simulink model "MVB1AnyLengthThree"  (R2013b)
settings: Solver=ode45  StartTime=0.0  StopTime=6e-5  RelTol=1e-3
libraries: simulink x4
(part 2 of 2)

== stateflow chart MVB1AnyLengthThree/MVB1/redundancy ==
  note: 从上一个接收事件后总线寂静1.4ms则产生一总线寂静的通知
  state Timer1 [parallel]
    settings: executionOrder=1
    state Timer
    state start
    state TimeOut
      entry:
      trust = false;
    Timer1.start -> Timer1.Timer : [judge(MFReceive1, MFReceive2, SFReceive1, SFReceive2, trust) == false]
        | {
        | t1 = clock_Counter;
        | }
    (default) -> Timer1.start
    Timer1.Timer -> Timer1.start [order 1] : [judge(MFReceive1, MFReceive2, SFReceive1, SFReceive2, trust) == true]
    Timer1.TimeOut -> Timer1.start
    Timer1.Timer -> Timer1.TimeOut [order 2] : [clock_Counter - t1 > (1400/prop) && judge(MFReceive1, MFReceive2, SFReceive1, SFReceive2, trust) == false]
  note: 上一个主帧接收后1.3ms没有收到主帧产生一个主帧超时的通知。
  state Timer2 [parallel]
    settings: executionOrder=2
    state Timer
    state start
    state TimeOut
      entry:
      trust = false;
    Timer2.start -> Timer2.Timer : [judge(MFReceive1, MFReceive2, trust) == true]
        | {
        | t1 = clock_Counter;
        | }
    (default) -> Timer2.start
    Timer2.Timer -> Timer2.start [order 1] : [judge(MFReceive1, MFReceive2,  trust) == true]
    Timer2.TimeOut -> Timer2.start
    Timer2.Timer -> Timer2.TimeOut [order 2] : [clock_Counter - t1 > (1300/prop) && judge(MFReceive1, MFReceive2,  trust) == false]
  note: 收到主帧后42.7us没有收到从帧产生从帧超时的通知。
  state Timer3 [parallel]
    settings: executionOrder=3
    state Timer
    state start
    state TimeOut
      entry:
      trust = false;
    Timer3.start -> Timer3.Timer : [judge(MFReceive1, MFReceive2, trust) == true]
        | {
        | t1 = clock_Counter;
        | }
    (default) -> Timer3.start
    Timer3.Timer -> Timer3.start [order 1] : [judge(SFReceive1, SFReceive2, trust) == true]
    Timer3.TimeOut -> Timer3.start
    Timer3.Timer -> Timer3.TimeOut [order 2] : [clock_Counter - t1 > (42.7/prop) && judge(SFReceive1, SFReceive2, trust) == false]
  note: 信任线未收到数据，而观察线收到数据时切换
  state observer [parallel]
    settings: executionOrder=4
    state A
      entry:
      trust = true;
    state B
      entry:
      trust = false;
    observer.A -> observer.B : [judge(MFReceive1, MFReceive2, SFReceive1, SFReceive2, trust) == false]
    (default) -> observer.A
    observer.B -> observer.A : [judge(MFReceive1, MFReceive2, SFReceive1, SFReceive2, trust) == true]
  state trans [parallel]
    settings: executionOrder=5
    state B
      during:
      MFReceive = MFReceive2;
      MFIn = MFIn2;
      SFReceive = SFReceive2;
      SFIn = SFIn2;
    state A
      during:
      MFReceive = MFReceive1;
      MFIn = MFIn1;
      SFReceive = SFReceive1;
      SFIn = SFIn1;
    trans.A -> trans.B : [trust == false]
        | {
        | MFReceive = MFReceive2;
        | MFIn = MFIn2;
        | SFReceive = SFReceive2;
        | SFIn = SFIn2;
        | }
    trans.B -> trans.A : [trust == true]
        | {
        | MFReceive = MFReceive1;
        | MFIn = MFIn1;
        | SFReceive = SFReceive1;
        | SFIn = SFIn1;
        | }
    (default) -> trans.A
  data: r function_output boolean; m1 function_input boolean; m2 function_input boolean; s1 function_input boolean; s2 function_input boolean; t function_input boolean; r function_output boolean; m1 function_input boolean; m2 function_input boolean; t function_input boolean; r function_output boolean; m1 function_input boolean; m2 function_input boolean; t function_input boolean; r function_output boolean; s1 function_input boolean; s2 function_input boolean; t function_input boolean; r function_output boolean; m1 function_input boolean; m2 function_input boolean; s1 function_input boolean; s2 function_input boolean; t function_input boolean; MFReceive1 input boolean; SFReceive1 input boolean; MFIn1 input uint32; SFIn1 input uint32; MFReceive2 input boolean; SFReceive2 input boolean; MFIn2 input uint32; SFIn2 input uint32; MFReceive output boolean; SFReceive output boolean; MFIn output uint32; SFIn output uint32; t1 local uint32; clock_Counter data_store_memory; trust local boolean =true; prop data_store_memory
  function r = judge(m1, m2, s1, s2, t):
    | function r = judge(m1, m2, s1, s2, t)
    | r = true;
    | if t == true
    |     if m1||s1 == false
    |         r = false;
    |     end
    | else
    |     if m2||s2 == false
    |         r = false;
    |     end
    | end
  function r = judge(m1, m2,t):
    | function r = judge(m1, m2,t)
    | r = false;
    | if t == true
    |     if m1 == true
    |         r = true;
    |     end
    | else
    |     if m2 == true
    |         r = true;
    |     end
    | end
  function r = judge(m1, m2, t):
    | function r = judge(m1, m2, t)
    | r = false;
    | if t == true
    |     if m1 == true
    |         r = true;
    |     end
    | else
    |     if m2 == true
    |         r = true;
    |     end
    | end
  function r = judgeSF(s1, s2, t):
    | function r = judgeSF(s1, s2, t)
    | r = false;
    | if t == true
    |     if s1 == true
    |         r = true;
    |     end
    | else
    |     if s2 == true
    |         r = true;
    |     end
    | end
  function r = judge(m1, m2, s1, s2, t):
    | function r = judge(m1, m2, s1, s2, t)
    | r = true;
    | if t == true
    |     if (m1||s1 == false) && (m2||s2 == true)
    |         r = false;
    |     end
    | else
    |     if (m2||s2 == false) && (m1||s1 == true)
    |         r = false;
    |     end
    | end

== stateflow chart MVB1AnyLengthThree/MVB3/Subsystem/Decoder ==
  state decodeSF
    decodeSF -> decodeSF [order 1] : CLK
        | {
        | ans = bitoperate.shiftbit(ans, 1) + SFIn;
        | count++;
        | }
  state bitoperate [group]
  state judge
    entry:
    ans = 0;
  state start
  state decodeMF
    decodeMF -> decodeMF [order 1] : CLK
        | {
        | ans = bitoperate.shiftbit(ans, 1) + MFIn;
        | count++;
        | }
  decodeSF -> judge [order 1] : [count==32]
      | {
      | SDataOut = ManchesterDecoding(ans);
      | count=0;
      | SFBuffer[SFBufferIndex] = SDataOut;
      | SFBufferIndex++;
      | }
  start -> decodeSF [order 2] : [SFInSign == true]
      | {
      | ans = 0;
      | count = 1;
      | SDataOut = 0;
      | ans = bitoperate.shiftbit(ans, 1) + SFIn;
      | SOutSign = true;
      | }
  judge -> decodeSF [order 1] : [SFInSign==true]
  judge -> start [order 2] : {
      | SOutSign = false;
      | SDataOut = 0;
      | }
  start -> decodeMF [order 1] : [MFInSign==true]
      | {
      | ans = 0;
      | count = 0;
      | MDataOut = 0;
      | MOutSign = true
      | ans = bitoperate.shiftbit(ans, 1) + MFIn;
      | count++;
      | }
  (default) -> start
  decodeMF -> start [order 1] : [count==32]
      | {
      | ans = ManchesterDecoding(ans);
      | MDataOut = ans;
      | MOutSign = false;
      | }
  data: num function_input uint32; r function_output uint32; data function_input uint32; num function_input uint32; r function_output uint32; r function_output uint32; data function_input uint32; MFIn input uint32; SFIn input uint32; MDataOut output uint32; MFInSign input boolean; count local uint32; SFInSign input boolean; SDataOut output uint32; MOutSign output boolean; SOutSign output boolean; ans local uint32; SFBuffer data_store_memory; SFBufferIndex data_store_memory
  events: CLK input EITHER_EDGE_EVENT
  function r = getbit(num):
    | function r = getbit(num)
    | r = bitget(num, 32);
  function r = shiftbit(data, num):
    | function r = shiftbit(data, num)
    | r = bitshift(data, num);
    | %for i=1:cnt
    | %   r = bitset(r, i, 0);
    | %end
  function r = ManchesterDecoding(data):
    | function r = ManchesterDecoding(data)
    | r = uint32(0);
    | for i = (1:2:32)
    |     x0 = bitget(data, i);
    |     x1 = bitget(data, i+1);
    |     if x0==0 && x1==1
    |         r = bitset(r, (i+1)/2, 1);
    |     else
    |         r = bitset(r, (i+1)/2, 0);
    |     end
    | end

== stateflow chart MVB1AnyLengthThree/MVB3/Subsystem/MainProc ==
  note: 上一个主帧接收后1.3ms没有收到主帧产生一个主帧超时的通知。
  state Timer [parallel]
    settings: executionOrder=1
    state Timer
      entry:
      t = clock_Counter;
      timeOut = false;
    state start
    state TimeOut
      entry:
      timeOut = true;
    start -> Timer.Timer : [startTimer == true]
    (default) -> start
    Timer.Timer -> start [order 1] : [endTimer == true]
    Timer.TimeOut -> start
    Timer.Timer -> Timer.TimeOut [order 2] : [clock_Counter - t > (1300/prop)]
  state mainproc [parallel]
    settings: executionOrder=2
    state StandbyEquip
      entry:
      startTimer = true;
      endTimer = false;
    state MainEquip
    state TimeOut
    state wait4ACT
    note: 等待其他设备返回ACT
    note: 等待其他设备返回OK，receiver在接收到OK以后立马放弃主权
    state TempEquip
      entry:
      startTimer = true;
      endTimer = false;
    (default) -> StandbyEquip
    mainproc.TimeOut -> StandbyEquip
    StandbyEquip -> mainproc.TimeOut [order 2] : [timeOut == true]
    TempEquip -> StandbyEquip [order 1] : [BA == false]
        | {
        | endTimer = true;
        | startTimer = false;
        | }
    StandbyEquip -> MainEquip [order 1] : [BA == true && ACT == true]
        | {
        | endTimer = true;
        | startTimer = false;
        | }
    MainEquip -> wait4ACT : [acceptACT == true]
        | {
        | t = clock_Counter;
        | }
    TempEquip -> mainproc.TimeOut [order 2] : [timeOut == true]
    wait4ACT -> TempEquip : [acceptDomain == true]
        | {
        | t = clock_Counter;
        | }
  data: BA data_store_memory; ACT local boolean =true; acceptACT data_store_memory; acceptDomain data_store_memory; t local uint32; clock_Counter data_store_memory; startTimer local boolean; timeOut local boolean; endTimer local boolean; prop data_store_memory

== stateflow chart MVB1AnyLengthThree/MVB2/Subsystem/Sender ==
  state SFSender [parallel]
    settings: executionOrder=1
    note: send**Signd的置位在接收到了请求数据的主帧后置位
    state sender [parallel]
      settings: executionOrder=1
      state wait
      state sendInfo
      state sendRandomSF
      state sendOK
      state transmission
        entry:
        SOutSign = true;
      (default) -> SFSender.sender.wait
      SFSender.sender.wait -> sendRandomSF [order 1] : [sendRandSFSign == true]
      SFSender.sender.wait -> sendOK [order 2] : [sendOkSign == true]
          | {
          | isMaster = true;
          | }
      SFSender.sender.wait -> sendInfo [order 3] : [sendACTSign == true]
      sendInfo -> SFSender.sender.transmission : {SFIndex = 1;
          | sendACTSign = false;}
      sendRandomSF -> SFSender.sender.transmission : {SFIndex = 0;
          | sendRandSFSign = false;}
      sendOK -> SFSender.sender.transmission : {SFIndex = 2;
          | sendOkSign = false;
          | init();
          | BA = true;
          | }
      SFSender.sender.transmission -> SFSender.sender : SFTransDone
          | {SDataOut = uint32(0);
          | SOutSign = false;
          | }
    state sendHolder [parallel]
      settings: executionOrder=2
      state judge
      state full
        SFSender.sendHolder.full -> SFSender.sendHolder.full [order 1] : CLK
            | {
            | SDataOut = bitoperate.getbit(input);
            | input = bitoperate.shiftbit(input, uint32(1));
            | count = count + 1;
            | }
      state empty
      judge -> SFSender.sendHolder.empty [order 2] : {
          | SOutSign = false;
          | SFCurrentIndex = 2;
          | send(SFTransDone, sender);
          | }
      SFSender.sendHolder.full -> judge [order 1] : [count == 32]
          | {
          | SFCurrentIndex = SFCurrentIndex + 1;
          | }
      judge -> SFSender.sendHolder.full [order 1] : [SFCurrentIndex <= SFT(SFIndex*16 + 1)]
          | {
          | input = ManchesterEncoding(uint32(SFT(SFIndex*16+SFCurrentIndex)));
          | count = 0;
          | }
      (default) -> SFSender.sendHolder.empty : {
          | SFCurrentIndex = 2;
          | }
      SFSender.sendHolder.empty -> SFSender.sendHolder.full : enter(sender.transmission)
          | {
          | input = ManchesterEncoding(uint32(SFT(SFIndex*16+SFCurrentIndex)));
          | SOutSign = true;
          | SDataOut = uint32(0);
          | count = 0;
          | }
  state MFSender [parallel]
    settings: executionOrder=2
    state sender [parallel]
      settings: executionOrder=1
      state sleep
      state wait
        entry:
        signal1 = true
      state transmission
        entry:
        signal1 = false;
        MOutSign = true;
        [acceptSF, acceptACT, acceptDomain] = setAcceptSignal(MFT(MFIndex));
      (default) -> sleep : {
          | init();
          | }
      sleep -> MFSender.sender.wait : CLK_3M
          | [BA==true ]
      MFSender.sender.transmission -> sleep : exit(buffer.full)
          | {
          | MDataOut = uint32(0);
          | MOutSign = false;
          | MFIndex = MFIndex + 1;
          | }
      MFSender.sender.wait -> MFSender.sender.transmission : [trans1 == true]
    state buffer [parallel]
      settings: executionOrder=2
      state full
        entry:
        count = 0;
        MFSender.buffer.full -> MFSender.buffer.full [order 1] : CLK
            | {
            | MDataOut = bitoperate.getbit(input);
            | input = bitoperate.shiftbit(input, uint32(1));
            | count = count + 1;
            | }
      state empty
      (default) -> MFSender.buffer.empty
      MFSender.buffer.full -> MFSender.buffer.empty [order 1] : [count == 32]
      MFSender.buffer.empty -> MFSender.buffer.full : enter(sender.transmission)
          | {
          | input =  ManchesterEncoding(MFT(MFIndex));
          | count = 0;
          | }
  state init [function]
    note: 请求随机从帧
        | 请求随机从帧
        | 请求2号的信息
        | 请求转移到2号
    note: SFT(1)代表随机的从帧
        | SFT(2)代表回复接受主权
        | SFT(3)代表回复设备ACT和BA
    (default) -> (junction 100) : {
        | BA = false;
        | MFIndex = 1;
        | isMaster = false;
        | SendSignal = false;
        | MFT(1) = getMF(0, 1);
        | MFT(2) = getMF(0, 3);
        | MFT(3) = getMF(8, 3);
        | MFT(4) = getMF(15, 3);
        | MFT(5) = 1;
        | SFT(1) = 4;
        | SFT(2) = 10894;
        | SFT(3) = 12428;
        | SFT(4) = 19;
        | SFT(17) = 4;
        | SFT(18) = 10894;
        | SFT(19) = 12832;
        | SFT(20) = 3;
        | SFT(33) = 4;
        | SFT(34) = 10894;
        | SFT(35) = 14464;
        | SFT(36) = 3;
        | clock_3M_shang = false;
        | sendRandSFSign = false;
        | sendACTSign = false;
        | sendRandSFSign = false;
        | }
  state bitoperate [group]
  (default) -> MFSender
  data: SFCurrentIndex local double; count local double; input local uint32; SFIndex local double; dataIn function_input uint32; SF function_output boolean; ACT function_output; Domain function_output; input local uint32; count local double; data function_input uint32; r function_output uint32; f_code function_input; addr function_input; r function_output; addr function_input; r function_output; r function_output uint32; data function_input uint32; num function_input uint32; r function_output uint32; data function_input uint32; num function_input uint32; r function_output uint32; MFReceive input boolean; MDataOut output uint32; clock_3M data_store_memory; clock_Counter data_store_memory; MFIndex local; MFT local uint32 size=5; trans1 data_store_memory; signal1 data_store_memory; SFReceive input boolean; sendOkSign data_store_memory; sendRandSFSign data_store_memory; sendACTSign data_store_memory; SDataOut output uint32; MOutSign output boolean; SOutSign output boolean; isMaster local boolean; acceptSF data_store_memory; BA data_store_memory; clock_3M_shang local boolean; acceptACT data_store_memory; acceptDomain data_store_memory; prop data_store_memory; SFT local uint16 size=100
  events: SFTransDone local FUNCTION_CALL_EVENT; CLK input EITHER_EDGE_EVENT; CLK_3M input EITHER_EDGE_EVENT
  function judgeMaster:
    | function judgeMaster
    | % 如果
    | if isMaster == true && SFIndex == 2
    |     isMaster = false;
    | end
  function [SF, ACT, Domain] = setAcceptSignal(dataIn):
    | function [SF, ACT, Domain] = setAcceptSignal(dataIn)
    | % 右移12位 仅保留帧头和fcode
    | dataInExAddr = bitshift(uint32(dataIn), -12);
    | % 先右移16位再左移4位 仅仅保留帧头
    | dataInStart = bitshift(bitshift(uint32(dataIn), -16), 4);
    | % 相减得到fcode
    | fcode = double(dataInExAddr - dataInStart);
    | SF = false;
    | Domain = false;
    | ACT = false;
    | if fcode == 0
    |     SF = true;
    | elseif fcode == 8
    |     ACT = true;
    | else
    |     Domain = true;
    | end
  function r = ManchesterEncoding(data):
    | function r = ManchesterEncoding(data)
    | r = data;
    | for i = 1:16
    |     x = bitget(data, i);
    |     if x == 0
    |         r = bitset(r, i*2-1, 1);
    |         r = bitset(r, i*2, 0);
    |     else
    |         r = bitset(r, i*2-1, 0);
    |         r = bitset(r, i*2, 1);
    |     end
    | end
  function r = getMF(f_code, addr):
    | function r = getMF(f_code, addr)
    | r = 3340042240;
    | r = r + bitshift(uint32(f_code), 12);
    | r = r + addr;
  function r = getSF(addr):
    | function r = getSF(addr)
    | r = 2833448960;
    | r = r + addr;
  function r = ManchesterDecoding(data):
    | function r = ManchesterDecoding(data)
    | r = uint32(0);
    | for i = (1:2:32)
    |     x0 = bitget(data, i);
    |     x1 = bitget(data, i+1);
    |     if x0==0 && x1==1
    |         r = bitset(r, (i+1)/2, 1);
    |     else
    |         r = bitset(r, (i+1)/2, 0);
    |     end
    | end
  function r = getbit(num):
    | function r = getbit(num)
    | r = bitget(num, 32);
  function r = shiftbit(data, num):
    | function r = shiftbit(data, num)
    | r = bitshift(data, num);
    | %for i=1:cnt
    | %   r = bitset(r, i, 0);
    | %end

== stateflow chart MVB1AnyLengthThree/MVB3/Subsystem/Receiver ==
  state receiveMF [parallel]
    settings: executionOrder=1
    state wait
    state wait4MFEnd
    state judgeAddr
    state MFReceive
    state MFcode0
    state MFcode8
    state MFcode15
    state MTrans
    (default) -> receiveMF.wait : {
        | t = clock_Counter;
        | }
    judgeAddr -> receiveMF.wait [order 2]
    MTrans -> receiveMF.wait : [sendRandSFSign == false && sendOkSign == false && sendACTSign == false]
        | {
        | t = clock_Counter;
        | }
    receiveMF.wait -> wait4MFEnd : [MFReceive==true]
    wait4MFEnd -> judgeAddr : [MFReceive == false]
        | {fcodeIn = uint8(getFCode(MFIn));
        | addrIn = uint16(getAddr(MFIn));
        | t = 0;
        | }
    judgeAddr -> MFReceive [order 1] : [addrIn == LogicAddr]
    MFReceive -> MFcode0 [order 2] : [fcodeIn == 0 && MFReceive == false ]
    MFReceive -> MFcode8 [order 3] : [fcodeIn == 8 && MFReceive == false]
    MFReceive -> MFcode15 [order 1] : [fcodeIn == 15 && MFReceive == false]
    MFcode0 -> MTrans : {sendRandSFSign = true}
    MFcode8 -> MTrans : {sendACTSign = true}
    MFcode15 -> MTrans : {sendOkSign = true}
  state receiveSF [parallel]
    settings: executionOrder=2
    note: acceptSF, acceptACT, acceptDomain在发送完主帧以后，根据主帧的类型进行相应的置位
        | 收到fcode为8的从帧之后，说明目标设备已经返回了OK，这时应该将ismaster设为1
    state wait
    state wait4SFEnd
    state judge4SF
    state wait4SF
    state wait4ACT
    state wait4Domain
    state STrans
    (default) -> receiveSF.wait
    (junction 96) -> receiveSF.wait : {
        | SFBufferIndex = 0;
        | initSFBuffer();
        | }
    receiveSF.wait -> wait4SFEnd : [SFReceive == true]
        | {
        | t = 0;
        | }
    wait4SFEnd -> judge4SF : [SFReceive == false]
    judge4SF -> (junction 96) [order 4]
    STrans -> (junction 96) : [SFReceive == false]
    judge4SF -> wait4Domain [order 3] : [acceptDomain == true]
    judge4SF -> wait4SF [order 1] : [acceptSF == true]
    judge4SF -> wait4ACT [order 2] : [acceptACT == true]
    wait4SF -> STrans : {
        | acceptSF = false;
        | }
    wait4ACT -> STrans : [getbit(SFBuffer[1], 6)]
        | {
        | acceptACT = false;
        | }
    wait4Domain -> STrans : [getbit(SFBuffer[1], 8) == 1]
        | {
        | acceptDomain = false;
        | BA = false;
        | }
  state initSFBuffer [function]
    (default) -> (junction 157) : /* init SFBuffer */
    (junction 149) -> (junction 151) [order 1] : [index<16]
    (junction 151) -> (junction 148) : {SFBuffer[index] = 0;}
    (junction 157) -> (junction 149) : {index=0;}
    (junction 148) -> (junction 149) : {index++;}
    (junction 149) -> (junction 145) [order 2]
  note: SFBufferIndex需要在每次读取后清零
  note: 期待目标设备返回OK
  data: index local double; dataIn function_input uint32; num function_input uint32; r function_output uint32; dataIn function_input double; r function_output double; data function_input uint32; r function_output uint32; dataIn function_input double; r function_output double; r function_output uint32; data function_input uint32; MFIn input uint32; SFIn input uint32; t local uint32; clock_Counter data_store_memory; clock_3M data_store_memory; MFReceive input boolean; SFReceive input boolean; fcodeIn local uint8; addrIn local uint16; trans1 data_store_memory; LogicAddr data_store_memory; sendRandSFSign data_store_memory; sendOkSign data_store_memory; sendACTSign data_store_memory; acceptSF data_store_memory; acceptDomain data_store_memory; acceptACT data_store_memory; BA data_store_memory; SFBuffer data_store_memory; SFBufferIndex data_store_memory
  function r = getbit(dataIn, num):
    | function r = getbit(dataIn, num)
    | r = bitget(uint32(dataIn), num);
  function r = getFCode(dataIn):
    | function r = getFCode(dataIn)
    | % 右移12位 仅保留帧头和fcode
    | dataInExAddr = bitshift(uint32(dataIn), -12);
    | % 先右移16位再左移4位 仅仅保留帧头
    | dataInStart = bitshift(bitshift(uint32(dataIn), -16), 4);
    | % 相减得到fcode
    | r = double(dataInExAddr - dataInStart);
  function r = ManchesterEncoding(data):
    | function r = ManchesterEncoding(data)
    | r = data;
    | for i = 1:16
    |     x = bitget(data, i);
    |     if x == 0
    |         r = bitset(r, i*2-1, 1);
    |         r = bitset(r, i*2, 0);
    |     else
    |         r = bitset(r, i*2-1, 0);
    |         r = bitset(r, i*2, 1);
    |     end
    | end
  function r = getAddr(dataIn):
    | function r = getAddr(dataIn)
    | % 把后12位也就是地址归零
    | dataInExAddr = bitshift(bitshift(uint32(dataIn), -12), 12);
    | % 相减获取地址
    | r = double(dataIn - dataInExAddr);
  function r = ManchesterDecoding(data):
    | function r = ManchesterDecoding(data)
    | r = uint32(0);
    | for i = (1:2:32)
    |     x0 = bitget(data, i);
    |     x1 = bitget(data, i+1);
    |     if x0==0 && x1==1
    |         r = bitset(r, (i+1)/2, 1);
    |     else
    |         r = bitset(r, (i+1)/2, 0);
    |     end
    | end

== stateflow chart MVB1AnyLengthThree/MVB3/Subsystem/Sender ==
  state SFSender [parallel]
    settings: executionOrder=1
    note: send**Signd的置位在接收到了请求数据的主帧后置位
    state sender [parallel]
      settings: executionOrder=1
      state wait
      state sendInfo
      state sendRandomSF
      state sendOK
      state transmission
        entry:
        SOutSign = true;
      (default) -> SFSender.sender.wait
      SFSender.sender.wait -> sendRandomSF [order 1] : [sendRandSFSign == true]
      SFSender.sender.wait -> sendOK [order 2] : [sendOkSign == true]
          | {
          | isMaster = true;
          | }
      SFSender.sender.wait -> sendInfo [order 3] : [sendACTSign == true]
      sendInfo -> SFSender.sender.transmission : {SFIndex = 1;
          | sendACTSign = false;}
      sendRandomSF -> SFSender.sender.transmission : {SFIndex = 0;
          | sendRandSFSign = false;}
      sendOK -> SFSender.sender.transmission : {SFIndex = 2;
          | sendOkSign = false;
          | init();
          | BA = true;
          | }
      SFSender.sender.transmission -> SFSender.sender : SFTransDone
          | {SDataOut = uint32(0);
          | SOutSign = false;
          | }
    state sendHolder [parallel]
      settings: executionOrder=2
      state judge
      state full
        SFSender.sendHolder.full -> SFSender.sendHolder.full [order 1] : CLK
            | {
            | SDataOut = bitoperate.getbit(input);
            | input = bitoperate.shiftbit(input, uint32(1));
            | count = count + 1;
            | }
      state empty
      judge -> SFSender.sendHolder.empty [order 2] : {
          | SOutSign = false;
          | SFCurrentIndex = 2;
          | send(SFTransDone, sender);
          | }
      SFSender.sendHolder.full -> judge [order 1] : [count == 32]
          | {
          | SFCurrentIndex = SFCurrentIndex + 1;
          | }
      judge -> SFSender.sendHolder.full [order 1] : [SFCurrentIndex <= SFT(SFIndex*16 + 1)]
          | {
          | input = ManchesterEncoding(uint32(SFT(SFIndex*16+SFCurrentIndex)));
          | count = 0;
          | }
      (default) -> SFSender.sendHolder.empty : {
          | SFCurrentIndex = 2;
          | }
      SFSender.sendHolder.empty -> SFSender.sendHolder.full : enter(sender.transmission)
          | {
          | input = ManchesterEncoding(uint32(SFT(SFIndex*16+SFCurrentIndex)));
          | SOutSign = true;
          | SDataOut = uint32(0);
          | count = 0;
          | }
  state MFSender [parallel]
    settings: executionOrder=2
    state sender [parallel]
      settings: executionOrder=1
      state sleep
      state wait
        entry:
        signal1 = true
      state transmission
        entry:
        signal1 = false;
        MOutSign = true;
        [acceptSF, acceptACT, acceptDomain] = setAcceptSignal(MFT(MFIndex));
      (default) -> sleep : {
          | init();
          | }
      sleep -> MFSender.sender.wait : CLK_3M
          | [BA==true]
      MFSender.sender.transmission -> sleep : exit(buffer.full)
          | {
          | MDataOut = uint32(0);
          | MOutSign = false;
          | MFIndex = MFIndex + 1;
          | }
      MFSender.sender.wait -> MFSender.sender.transmission : [trans1 == true]
    state buffer [parallel]
      settings: executionOrder=2
      state full
        entry:
        count = 0;
        MFSender.buffer.full -> MFSender.buffer.full [order 1] : CLK
            | {
            | MDataOut = bitoperate.getbit(input);
            | input = bitoperate.shiftbit(input, uint32(1));
            | count = count + 1;
            | }
      state empty
      (default) -> MFSender.buffer.empty
      MFSender.buffer.full -> MFSender.buffer.empty [order 1] : [count == 32]
      MFSender.buffer.empty -> MFSender.buffer.full : enter(sender.transmission)
          | {
          | input =  ManchesterEncoding(MFT(MFIndex));
          | count = 0;
          | }
  state init [function]
    note: 请求随机从帧
        | 请求随机从帧
        | 请求2号的信息
        | 请求转移到2号
    note: SFT(1)代表随机的从帧
        | SFT(2)代表回复接受主权
        | SFT(3)代表回复设备ACT和BA
    (default) -> (junction 100) : {
        | BA = false;
        | MFIndex = 1;
        | isMaster = false;
        | SendSignal = false;
        | MFT(1) = getMF(0, 1);
        | MFT(2) = getMF(0, 2);
        | MFT(3) = getMF(8, 1);
        | MFT(4) = getMF(15, 1);
        | MFT(5) = 1;
        | SFT(1) = 4;
        | SFT(2) = 10894;
        | SFT(3) = 12428;
        | SFT(4) = 19;
        | SFT(17) = 4;
        | SFT(18) = 10894;
        | SFT(19) = 12832;
        | SFT(20) = 3;
        | SFT(33) = 4;
        | SFT(34) = 10894;
        | SFT(35) = 14464;
        | SFT(36) = 3;
        | clock_3M_shang = false;
        | sendRandSFSign = false;
        | sendACTSign = false;
        | sendRandSFSign = false;
        | }
  state bitoperate [group]
  (default) -> MFSender
  data: SFCurrentIndex local double; count local double; input local uint32; SFIndex local double; dataIn function_input uint32; SF function_output boolean; ACT function_output; Domain function_output; input local uint32; count local double; data function_input uint32; r function_output uint32; f_code function_input; addr function_input; r function_output; addr function_input; r function_output; r function_output uint32; data function_input uint32; num function_input uint32; r function_output uint32; data function_input uint32; num function_input uint32; r function_output uint32; MFReceive input boolean; MDataOut output uint32; clock_3M data_store_memory; clock_Counter data_store_memory; MFIndex local; MFT local uint32 size=5; trans1 data_store_memory; signal1 data_store_memory; SFReceive input boolean; sendOkSign data_store_memory; sendRandSFSign data_store_memory; sendACTSign data_store_memory; SDataOut output uint32; MOutSign output boolean; SOutSign output boolean; isMaster local boolean; acceptSF data_store_memory; BA data_store_memory; clock_3M_shang local boolean; acceptACT data_store_memory; acceptDomain data_store_memory; prop data_store_memory; SFT local uint16 size=100
  events: SFTransDone local FUNCTION_CALL_EVENT; CLK input EITHER_EDGE_EVENT; CLK_3M input EITHER_EDGE_EVENT
  function judgeMaster:
    | function judgeMaster
    | % 如果
    | if isMaster == true && SFIndex == 2
    |     isMaster = false;
    | end
  function [SF, ACT, Domain] = setAcceptSignal(dataIn):
    | function [SF, ACT, Domain] = setAcceptSignal(dataIn)
    | % 右移12位 仅保留帧头和fcode
    | dataInExAddr = bitshift(uint32(dataIn), -12);
    | % 先右移16位再左移4位 仅仅保留帧头
    | dataInStart = bitshift(bitshift(uint32(dataIn), -16), 4);
    | % 相减得到fcode
    | fcode = double(dataInExAddr - dataInStart);
    | SF = false;
    | Domain = false;
    | ACT = false;
    | if fcode == 0
    |     SF = true;
    | elseif fcode == 8
    |     ACT = true;
    | else
    |     Domain = true;
    | end
  function r = ManchesterEncoding(data):
    | function r = ManchesterEncoding(data)
    | r = data;
    | for i = 1:16
    |     x = bitget(data, i);
    |     if x == 0
    |         r = bitset(r, i*2-1, 1);
    |         r = bitset(r, i*2, 0);
    |     else
    |         r = bitset(r, i*2-1, 0);
    |         r = bitset(r, i*2, 1);
    |     end
    | end
  function r = getMF(f_code, addr):
    | function r = getMF(f_code, addr)
    | r = 3340042240;
    | r = r + bitshift(uint32(f_code), 12);
    | r = r + addr;
  function r = getSF(addr):
    | function r = getSF(addr)
    | r = 2833448960;
    | r = r + addr;
  function r = ManchesterDecoding(data):
    | function r = ManchesterDecoding(data)
    | r = uint32(0);
    | for i = (1:2:32)
    |     x0 = bitget(data, i);
    |     x1 = bitget(data, i+1);
    |     if x0==0 && x1==1
    |         r = bitset(r, (i+1)/2, 1);
    |     else
    |         r = bitset(r, (i+1)/2, 0);
    |     end
    | end
  function r = getbit(num):
    | function r = getbit(num)
    | r = bitget(num, 32);
  function r = shiftbit(data, num):
    | function r = shiftbit(data, num)
    | r = bitshift(data, num);
    | %for i=1:cnt
    | %   r = bitset(r, i, 0);
    | %end

== stateflow chart MVB1AnyLengthThree/MVB2/redundancy ==
  note: 从上一个接收事件后总线寂静1.4ms则产生一总线寂静的通知
  state Timer1 [parallel]
    settings: executionOrder=1
    state Timer
    state start
    state TimeOut
      entry:
      trust = false;
    Timer1.start -> Timer1.Timer : [judge(MFReceive1, MFReceive2, SFReceive1, SFReceive2, trust) == false]
        | {
        | t1 = clock_Counter;
        | }
    (default) -> Timer1.start
    Timer1.Timer -> Timer1.start [order 1] : [judge(MFReceive1, MFReceive2, SFReceive1, SFReceive2, trust) == true]
    Timer1.TimeOut -> Timer1.start
    Timer1.Timer -> Timer1.TimeOut [order 2] : [clock_Counter - t1 > (1400/prop) && judge(MFReceive1, MFReceive2, SFReceive1, SFReceive2, trust) == false]
  note: 上一个主帧接收后1.3ms没有收到主帧产生一个主帧超时的通知。
  state Timer2 [parallel]
    settings: executionOrder=2
    state Timer
    state start
    state TimeOut
      entry:
      trust = false;
    Timer2.start -> Timer2.Timer : [judge(MFReceive1, MFReceive2, trust) == true]
        | {
        | t1 = clock_Counter;
        | }
    (default) -> Timer2.start
    Timer2.Timer -> Timer2.start [order 1] : [judge(MFReceive1, MFReceive2,  trust) == true]
    Timer2.TimeOut -> Timer2.start
    Timer2.Timer -> Timer2.TimeOut [order 2] : [clock_Counter - t1 > (1300/prop) && judge(MFReceive1, MFReceive2,  trust) == false]
  note: 收到主帧后42.7us没有收到从帧产生从帧超时的通知。
  state Timer3 [parallel]
    settings: executionOrder=3
    state Timer
    state start
    state TimeOut
      entry:
      trust = false;
    Timer3.start -> Timer3.Timer : [judge(MFReceive1, MFReceive2, trust) == true]
        | {
        | t1 = clock_Counter;
        | }
    (default) -> Timer3.start
    Timer3.Timer -> Timer3.start [order 1] : [judge(SFReceive1, SFReceive2, trust) == true]
    Timer3.TimeOut -> Timer3.start
    Timer3.Timer -> Timer3.TimeOut [order 2] : [clock_Counter - t1 > (42.7/prop) && judge(SFReceive1, SFReceive2, trust) == false]
  note: 信任线未收到数据，而观察线收到数据时切换
  state observer [parallel]
    settings: executionOrder=4
    state A
      entry:
      trust = true;
    state B
      entry:
      trust = false;
    observer.A -> observer.B : [judge(MFReceive1, MFReceive2, SFReceive1, SFReceive2, trust) == false]
    (default) -> observer.A
    observer.B -> observer.A : [judge(MFReceive1, MFReceive2, SFReceive1, SFReceive2, trust) == true]
  state trans [parallel]
    settings: executionOrder=5
    state B
      during:
      MFReceive = MFReceive2;
      MFIn = MFIn2;
      SFReceive = SFReceive2;
      SFIn = SFIn2;
    state A
      during:
      MFReceive = MFReceive1;
      MFIn = MFIn1;
      SFReceive = SFReceive1;
      SFIn = SFIn1;
    trans.A -> trans.B : [trust == false]
        | {
        | MFReceive = MFReceive2;
        | MFIn = MFIn2;
        | SFReceive = SFReceive2;
        | SFIn = SFIn2;
        | }
    trans.B -> trans.A : [trust == true]
        | {
        | MFReceive = MFReceive1;
        | MFIn = MFIn1;
        | SFReceive = SFReceive1;
        | SFIn = SFIn1;
        | }
    (default) -> trans.A
  data: r function_output boolean; m1 function_input boolean; m2 function_input boolean; s1 function_input boolean; s2 function_input boolean; t function_input boolean; r function_output boolean; m1 function_input boolean; m2 function_input boolean; t function_input boolean; r function_output boolean; m1 function_input boolean; m2 function_input boolean; t function_input boolean; r function_output boolean; s1 function_input boolean; s2 function_input boolean; t function_input boolean; r function_output boolean; m1 function_input boolean; m2 function_input boolean; s1 function_input boolean; s2 function_input boolean; t function_input boolean; MFReceive1 input boolean; SFReceive1 input boolean; MFIn1 input uint32; SFIn1 input uint32; MFReceive2 input boolean; SFReceive2 input boolean; MFIn2 input uint32; SFIn2 input uint32; MFReceive output boolean; SFReceive output boolean; MFIn output uint32; SFIn output uint32; t1 local uint32; clock_Counter data_store_memory; trust local boolean =true; prop data_store_memory
  function r = judge(m1, m2, s1, s2, t):
    | function r = judge(m1, m2, s1, s2, t)
    | r = true;
    | if t == true
    |     if m1||s1 == false
    |         r = false;
    |     end
    | else
    |     if m2||s2 == false
    |         r = false;
    |     end
    | end
  function r = judge(m1, m2,t):
    | function r = judge(m1, m2,t)
    | r = false;
    | if t == true
    |     if m1 == true
    |         r = true;
    |     end
    | else
    |     if m2 == true
    |         r = true;
    |     end
    | end
  function r = judge(m1, m2, t):
    | function r = judge(m1, m2, t)
    | r = false;
    | if t == true
    |     if m1 == true
    |         r = true;
    |     end
    | else
    |     if m2 == true
    |         r = true;
    |     end
    | end
  function r = judgeSF(s1, s2, t):
    | function r = judgeSF(s1, s2, t)
    | r = false;
    | if t == true
    |     if s1 == true
    |         r = true;
    |     end
    | else
    |     if s2 == true
    |         r = true;
    |     end
    | end
  function r = judge(m1, m2, s1, s2, t):
    | function r = judge(m1, m2, s1, s2, t)
    | r = true;
    | if t == true
    |     if (m1||s1 == false) && (m2||s2 == true)
    |         r = false;
    |     end
    | else
    |     if (m2||s2 == false) && (m1||s1 == true)
    |         r = false;
    |     end
    | end

== stateflow chart MVB1AnyLengthThree/MVB3/redundancy ==
  note: 从上一个接收事件后总线寂静1.4ms则产生一总线寂静的通知
  state Timer1 [parallel]
    settings: executionOrder=1
    state Timer
    state start
    state TimeOut
      entry:
      trust = false;
    Timer1.start -> Timer1.Timer : [judge(MFReceive1, MFReceive2, SFReceive1, SFReceive2, trust) == false]
        | {
        | t1 = clock_Counter;
        | }
    (default) -> Timer1.start
    Timer1.Timer -> Timer1.start [order 1] : [judge(MFReceive1, MFReceive2, SFReceive1, SFReceive2, trust) == true]
    Timer1.TimeOut -> Timer1.start
    Timer1.Timer -> Timer1.TimeOut [order 2] : [clock_Counter - t1 > (1400/prop) && judge(MFReceive1, MFReceive2, SFReceive1, SFReceive2, trust) == false]
  note: 上一个主帧接收后1.3ms没有收到主帧产生一个主帧超时的通知。
  state Timer2 [parallel]
    settings: executionOrder=2
    state Timer
    state start
    state TimeOut
      entry:
      trust = false;
    Timer2.start -> Timer2.Timer : [judge(MFReceive1, MFReceive2, trust) == true]
        | {
        | t1 = clock_Counter;
        | }
    (default) -> Timer2.start
    Timer2.Timer -> Timer2.start [order 1] : [judge(MFReceive1, MFReceive2,  trust) == true]
    Timer2.TimeOut -> Timer2.start
    Timer2.Timer -> Timer2.TimeOut [order 2] : [clock_Counter - t1 > (1300/prop) && judge(MFReceive1, MFReceive2,  trust) == false]
  note: 收到主帧后42.7us没有收到从帧产生从帧超时的通知。
  state Timer3 [parallel]
    settings: executionOrder=3
    state Timer
    state start
    state TimeOut
      entry:
      trust = false;
    Timer3.start -> Timer3.Timer : [judge(MFReceive1, MFReceive2, trust) == true]
        | {
        | t1 = clock_Counter;
        | }
    (default) -> Timer3.start
    Timer3.Timer -> Timer3.start [order 1] : [judge(SFReceive1, SFReceive2, trust) == true]
    Timer3.TimeOut -> Timer3.start
    Timer3.Timer -> Timer3.TimeOut [order 2] : [clock_Counter - t1 > (42.7/prop) && judge(SFReceive1, SFReceive2, trust) == false]
  note: 信任线未收到数据，而观察线收到数据时切换
  state observer [parallel]
    settings: executionOrder=4
    state A
      entry:
      trust = true;
    state B
      entry:
      trust = false;
    observer.A -> observer.B : [judge(MFReceive1, MFReceive2, SFReceive1, SFReceive2, trust) == false]
    (default) -> observer.A
    observer.B -> observer.A : [judge(MFReceive1, MFReceive2, SFReceive1, SFReceive2, trust) == true]
  state trans [parallel]
    settings: executionOrder=5
    state B
      during:
      MFReceive = MFReceive2;
      MFIn = MFIn2;
      SFReceive = SFReceive2;
      SFIn = SFIn2;
    state A
      during:
      MFReceive = MFReceive1;
      MFIn = MFIn1;
      SFReceive = SFReceive1;
      SFIn = SFIn1;
    trans.A -> trans.B : [trust == false]
        | {
        | MFReceive = MFReceive2;
        | MFIn = MFIn2;
        | SFReceive = SFReceive2;
        | SFIn = SFIn2;
        | }
    trans.B -> trans.A : [trust == true]
        | {
        | MFReceive = MFReceive1;
        | MFIn = MFIn1;
        | SFReceive = SFReceive1;
        | SFIn = SFIn1;
        | }
    (default) -> trans.A
  data: r function_output boolean; m1 function_input boolean; m2 function_input boolean; s1 function_input boolean; s2 function_input boolean; t function_input boolean; r function_output boolean; m1 function_input boolean; m2 function_input boolean; t function_input boolean; r function_output boolean; m1 function_input boolean; m2 function_input boolean; t function_input boolean; r function_output boolean; s1 function_input boolean; s2 function_input boolean; t function_input boolean; r function_output boolean; m1 function_input boolean; m2 function_input boolean; s1 function_input boolean; s2 function_input boolean; t function_input boolean; MFReceive1 input boolean; SFReceive1 input boolean; MFIn1 input uint32; SFIn1 input uint32; MFReceive2 input boolean; SFReceive2 input boolean; MFIn2 input uint32; SFIn2 input uint32; MFReceive output boolean; SFReceive output boolean; MFIn output uint32; SFIn output uint32; t1 local uint32; clock_Counter data_store_memory; trust local boolean =true; prop data_store_memory
  function r = judge(m1, m2, s1, s2, t):
    | function r = judge(m1, m2, s1, s2, t)
    | r = true;
    | if t == true
    |     if m1||s1 == false
    |         r = false;
    |     end
    | else
    |     if m2||s2 == false
    |         r = false;
    |     end
    | end
  function r = judge(m1, m2,t):
    | function r = judge(m1, m2,t)
    | r = false;
    | if t == true
    |     if m1 == true
    |         r = true;
    |     end
    | else
    |     if m2 == true
    |         r = true;
    |     end
    | end
  function r = judge(m1, m2, t):
    | function r = judge(m1, m2, t)
    | r = false;
    | if t == true
    |     if m1 == true
    |         r = true;
    |     end
    | else
    |     if m2 == true
    |         r = true;
    |     end
    | end
  function r = judgeSF(s1, s2, t):
    | function r = judgeSF(s1, s2, t)
    | r = false;
    | if t == true
    |     if s1 == true
    |         r = true;
    |     end
    | else
    |     if s2 == true
    |         r = true;
    |     end
    | end
  function r = judge(m1, m2, s1, s2, t):
    | function r = judge(m1, m2, s1, s2, t)
    | r = true;
    | if t == true
    |     if (m1||s1 == false) && (m2||s2 == true)
    |         r = false;
    |     end
    | else
    |     if (m2||s2 == false) && (m1||s1 == true)
    |         r = false;
    |     end
    | end

== stateflow chart MVB1AnyLengthThree/Timer/Chart ==
  state trans
    during:
    dataOut = dataIn;
  (default) -> trans
  data: dataIn input double; dataOut output double
